simulink model "Model_grzalka_wentylator"  (R2017b)
settings: Solver=ode4  StartTime=0.0  StopTime=30  FixedStep=0.01  RelTol=1e-3
undefined symbols (not defined in the file): A, B, C, D, F
libraries: slident x1
settings Model: Creator=SaDiablo  LastModifiedBy=SaDiablo

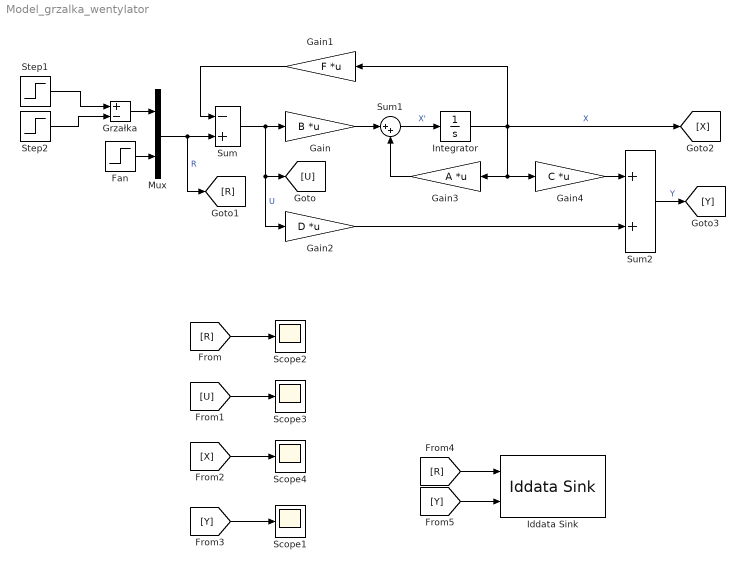
== system Model_grzalka_wentylator ==
  Fan : Step  Time=0  SampleTime=0.01
  Gain : Gain  Gain=B  Multiplication=Matrix(K*u) (u vector)
  Gain1 : Gain  Gain=F  Multiplication=Matrix(K*u) (u vector)
  Gain2 : Gain  Gain=D  Multiplication=Matrix(K*u) (u vector)
  Gain3 : Gain  Gain=A  Multiplication=Matrix(K*u) (u vector)
  Gain4 : Gain  Gain=C  Multiplication=Matrix(K*u) (u vector)
  Grzałka : Sum  Inputs=+-
  Iddata Sink : slident/Iddata Sink  datasetname=data  Ts=0.01  isu=on  isy=on
      settings: SourceProductName=System Identification Toolbox  SourceProductBaseCode=ID
  Integrator : Integrator
  Mux : Mux  Inputs=2
  Scope{1..4} (4 alike) : Scope
  Step1 : Step  Time=5  SampleTime=0.01
  Step2 : Step  Time=7  SampleTime=0.01
  Sum : Sum  Inputs=-+
  Sum1 : Sum  Inputs=|++
  Sum2 : Sum
  wires:
  Step1/1 -> Grzałka/1
  Step2/1 -> Grzałka/2
  Grzałka/1 -> Mux/1
  Fan/1 -> Mux/2
  Mux/1 -> [R], Sum/2  "R"
  Sum/1 -> [U], Gain2/1, Gain/1  "U"
  Gain/1 -> Sum1/1
  Sum1/1 -> Integrator/1  "X'"
  Gain3/1 -> Sum1/2
  Integrator/1 -> Gain4/1, Gain3/1, [X], Gain1/1  "X"
  Gain1/1 -> Sum/1
  Gain4/1 -> Sum2/1
  Gain2/1 -> Sum2/2
  Sum2/1 -> [Y]  "Y"
  [R] -> Scope2/1
  [U] -> Scope3/1
  [X] -> Scope4/1
  [Y] -> Scope1/1
  [Y] -> Iddata Sink/2
  [R] -> Iddata Sink/1
